simulink model "my_hdlcoder_sqrt_bitset_control"  (R2024a)
settings: Solver=VariableStepAuto  StartTime=0.0  StopTime=stoptime  RelTol=1e-3
libraries: dspsrcs4 x1, HDLMathLib x1
settings Model: Creator=lingg  LastModifiedBy=lingg
settings DataIOCC: SaveOutput=off  SignalLogging=off  SaveTime=off  ReturnWorkspaceOutputs=off
settings OptimizationCC: BlockReduction=off  ConditionallyExecuteInputs=off
settings DebuggingCC: IntegerOverflowMsg=none  IntegerSaturationMsg=none

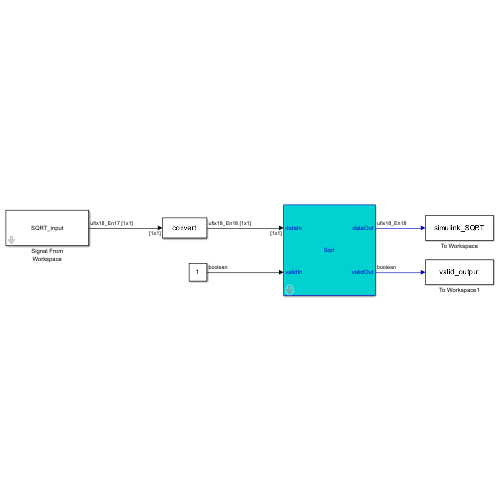
[thumbnail: Simulink's stored preview of the top-level diagram]
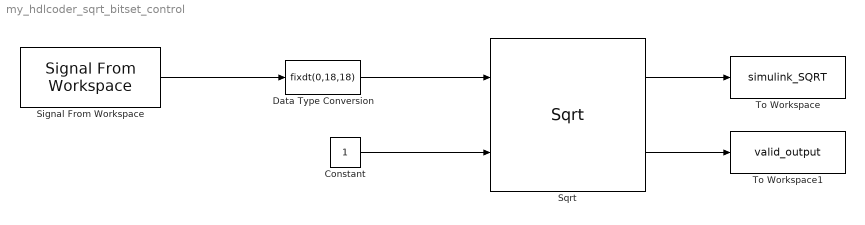
== system my_hdlcoder_sqrt_bitset_control ==
  Constant : Constant  OutDataTypeStr=boolean  SampleTime=-1
  Data Type Conversion : DataTypeConversion  OutDataTypeStr=fixdt(0,18,18)  RndMeth=Floor
  Signal From Workspace : dspsrcs4/Signal From Workspace  X=SQRT_input  Ts=1  nsamps=1  OutputAfterFinalValue=Setting to zero  ignoreOrWarnInputAndFrameLengths=off  OutputFrames=off
  Sqrt : HDLMathLib/Sqrt  latencyMode=Max  customLatencyValue=0  SaturateOnIntegerOverflow=on
  To Workspace : ToWorkspace  VariableName=simulink_SQRT  SampleTime=-1
      settings: Save2DSignal=2-D array (concatenate along first dimension)
  To Workspace1 : ToWorkspace  VariableName=valid_output  SampleTime=-1
      settings: Save2DSignal=2-D array (concatenate along first dimension)
  wires:
  Signal From Workspace/1 -> Data Type Conversion/1
  Data Type Conversion/1 -> Sqrt/1
  Constant/1 -> Sqrt/2
  Sqrt/1 -> To Workspace/1
  Sqrt/2 -> To Workspace1/1
